simulink model "fsmtest"  (R2020b)
settings: Solver=FixedStepAuto  StartTime=0.0  StopTime=inf  RelTol=1e-3  EnableMultiTasking=on
libraries: arduinolib x1, arduinowifilib x1
settings Model: SILPILModeSetting=veronly  ExtModeTrigDuration=2  Creator=Ege  LastModifiedBy=Ege
settings OptimizationCC: EnhancedBackFolding=on  PassReuseOutputArgsAs=Individual arguments  ZeroExternalMemoryAtStartup=off  ZeroInternalMemoryAtStartup=off  MaxStackSize=64  OptimizeBlockOrder=speed  DifferentSizesBufferReuse=on  OptimizationCustomize=off  EfficientTunableParamExpr=on
settings DebuggingCC: ParameterTunabilityLossMsg=error
settings HardwareCC: ProdBitPerPointer=32  ProdBitPerSizeT=32  ProdBitPerPtrDiffT=32  ProdLargestAtomicInteger=Long  ProdLargestAtomicFloat=Double  ProdWordSize=32  ProdHWDeviceType=ARM Compatible->ARM Cortex
settings SFSimCC: MATLABDynamicMemAlloc=off
settings RTWCC: Description=Embedded Coder  SystemTargetFile=ert.tlc  HardwareBoard=Arduino Nano 33 IoT  TemplateMakefile=ert_default_tmf  Toolchain=Arduino ARM  BuildConfiguration=Faster Runs
settings CodeAppCC: ForceParamTrailComments=on  IgnoreCustomStorageClasses=off  OperatorAnnotations=on  SimulinkDataObjDesc=on  SFDataObjDesc=on  InsertBlockDesc=on
settings ERTTargetCC: SupportContinuousTime=on  SupportVariableSizeSignals=on  ExtModeTransport=3  ExtModeStaticAllocSize=8192  ExtModeMexFile=ext_xcp  ExtModeIntrfLevel=Level2 - Open

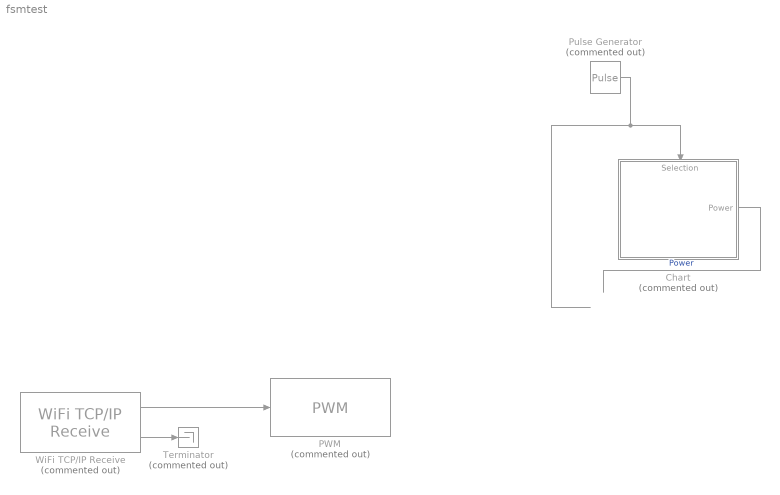
== system fsmtest ==
  Chart : Stateflow chart  Commented=on  TreatAsAtomicUnit=on
      settings: PortSchema="{\"entries\":[{\"content\":{\"sides\":[{\"content\":{\"connectorIds\":[]},\"type\":\"ConnectorPlacement.EquallySpacedRectSide\",\"uuid\":\"4780532d-0514-40f4-b258-38ecf4521520\"},{\"content\":{\"connectorIds\":[\"Out1\"],\"side\":\"RIGHT\"},\"type\":\"ConnectorPlacement.EquallySpacedRectSide\",\"uuid\":\"81295485-ee17-4df1-9b00-c017ae5f544b\"},{\"content\":{\"connectorIds\":[\"In1\"],\"side\":\"TOP\"},\"type\":\"ConnectorPlacement.EquallySpacedRectSide\",\"uuid\":\"68b487fb-56b0-41e6-8c22-1b2290b8b9df\"},{\"content\":{\"connectorIds\":[],\"side\":\"BOTTOM\"},\"type\":\"ConnectorPlacement.EquallySpacedRectSide\",\"uuid\":\"605eac78-1c86-4cb3-b2e7-d005bdc1f880\"},{\"content\":{\"connectorIds\":[],\"side\":\"HIDDEN\"},\"type\":\"ConnectorPlacement.EquallySpacedRectSide\",\"uuid\":\"5177aa4b-a8e4-4df7-8d95-e02c5ee9ca46\"}]},\"type\":\"ConnectorPlacement.EquallySpacedConnector\",\"uuid\":\"12a00e08-d74b-48d0-bf46-5de96b83edcf\"}],\"packageUris\":[\"http://schema.mathworks.com/mf0/Connector/R2020b\"],\"version\":\"1.0\"}"
  PWM : arduinolib/PWM  Commented=on  pinNumber=9  frequencyType=Default  desiredFrequency=490.2  achievableFrequency=490.2
  Pulse Generator : DiscretePulseGenerator  Commented=on  PulseType=Time based  Period=6  PulseWidth=10  PhaseDelay=1
  Terminator : Terminator  Commented=on
  WiFi TCP/IP Receive : arduinowifilib/WiFi TCP//IP Receive  Commented=on  Mode_=Server  serverport=25000  RemoteAddr_=192.168.1.2  RemoteServerPort_=25000  DataType_=uint8  DataSize_=1  SampleTime_=0.1  remoteipoctet1=192  remoteipoctet2=168  remoteipoctet3=1  remoteipoctet4=2  wifiTCPServerIndex=0  wifiTCPClientIndex=0  blockPlatform=ARDUINO  isARMArch=true  SimulateUsing=Code generation  BlockingMode_=off  BlockTimeout_=0.1
      settings: SourceProductBaseCode=ARDUINO
  wires:
  Pulse Generator/1 -> Chart/1(Selection)
  Chart/1(Power) -> ?  "Power"
  WiFi TCP/IP Receive/2 -> Terminator/1
  WiFi TCP/IP Receive/1 -> PWM/1

== stateflow chart fsmtest/Chart ==
  state Init
  state Off
    en:
    Power:0;
  state On
    en:
    Power = 1;
  (default) -> Init : {Power=0}
  Off -> Init
  Init -> On : [Selection == 1]
  On -> Off : after(4,sec)
  data: Selection input =1; Power output double
